simulink model "test"  (R2015b)
settings: Solver=VariableStepAuto  StartTime=0.0  StopTime=2000  RelTol=1e-3
settings Model: Creator=rajiv  LastModifiedBy=rajiv

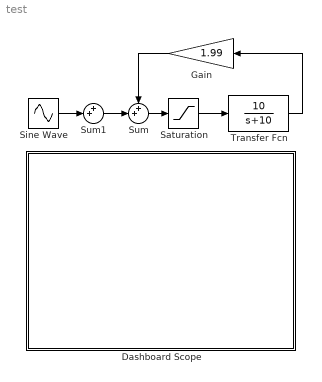
== system test ==
  Dashboard Scope : Subsystem  DialogController=hmiCreateDDGDialog  IsWebBlock=on  mask(MWDashboardBlock){webBlockId=4353073f-cf43-49d2-95a7-c96afbc2a60d, webBlockType=sdiscope, ShowInitialText=on, HMISrcModelName=test}
      mask prompts: webBlockId "WebBlock Id"; webBlockType "WebBlock Type"; HMISrcModelName "Source Model"
      mask Help: helpview([docroot '/mapfiles/simulink.map'], 'hmi_scope')
      mask Display:
      | if strcmp(get_param(bdroot(gcb),'BlockDiagramType'), 'library')
      |     image([(matlabroot) '/toolbox/simulink/hmi/icons/DashboardScope.png']);
      | end
  Gain : Gain  Gain=1.99
  Saturation : Saturate  UpperLimit=1  LowerLimit=-1
  Sine Wave : Sin  Frequency=.01  SampleTime=0
  Sum : Sum  Inputs=++|
  Sum1 : Sum  Inputs=++|
  Transfer Fcn : TransferFcn  Numerator=[10]  Denominator=[1 10]
  wires:
  Saturation/1 -> Transfer Fcn/1
  Gain/1 -> Sum/1
  Sum/1 -> Saturation/1
  Transfer Fcn/1 -> Gain/1
  Sum1/1 -> Sum/2
  Sine Wave/1 -> Sum1/2

== system test/Dashboard Scope ==
